simulink model "bataryatermaletkisiz"  (R2020a)
settings: Solver=VariableStepAuto  StartTime=0.0  StopTime=10.0  RelTol=1e-3
undefined symbols (not defined in the file): Ion, Lithium
libraries: electricdrivelib x34, powerlib x5
settings Model: Creator=ASUS  LastModifiedBy=ASUS

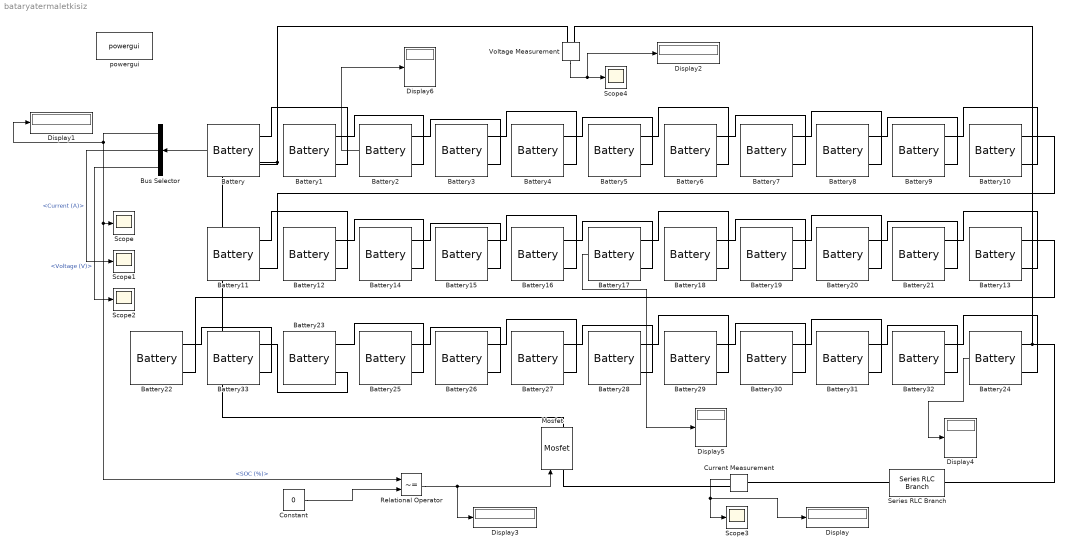
== system bataryatermaletkisiz ==
  Battery{,1..33} (34 alike) : electricdrivelib/Extra Sources/Battery  BatType=Lithium-Ion  ShowTempParam=off  ThermalPreset=no  ShowAgeParam=off  NomV=3.6  NomQ=40.2  SOC=90  Batt_Tr=30  PresetModel=on  MaxQ=40.2  MinV=2.7  FullV=4.1904  Dis_rate=17.4783  R=0.00089552  Normal_OP=36.3548  expZone="[3.8894       1.975]"  current=[6.5 13 32.5]  Units=Time  Tci=20  NomT=20  T2=-30  MaxQ2=4.8  FullV2=7.1  Normal_OP2=5.655  expZone2="[6.58           1]"  Rca=0.6  ti=2000  Dp=0  Neq0=0  Tsim=1e6  Ta1=25  Qeol=5.4*0.9  Reol=0.013333*1.2  Char_age=[2.3478, 3]  Dis_age=[2.3478, 10]  N1=1500  N2=10500  N3=1000  N4=1400  Ta2=45  N5=950
  Bus Selector : BusSelector  OutputSignals=SOC (%),Current (A),Voltage (V)
  Constant : Constant  Value=0
  Current Measurement : powerlib/Measurements/Current Measurement  PhasorSimulation=off  OutputType=Complex  PSBequivalent=0
  Display{,1..6} (7 alike) : Display
  Mosfet : powerlib/Power Electronics/Mosfet  Ron=0.1  Lon=0  Rd=0.01  Vfd=0  IC=0  Rs=1e5  Cs=inf  Measurements=on
  Relational Operator : RelationalOperator  Operator=~=  OutDataTypeStr=boolean  RndMeth=Simplest
  Scope{,1..4} (5 alike) : Scope
  Series RLC Branch : powerlib/Elements/Series RLC Branch  LConnTagsString=__new0  RConnTagsString=__new0  BranchType=R  Resistance=48.4  Inductance=1e-3  SetiL0=off  InitialCurrent=0  Capacitance=1e-6  Setx0=off  InitialVoltage=0  Measurements=None
  Voltage Measurement : powerlib/Measurements/Voltage Measurement  PhasorSimulation=off  OutputType=Complex  PSBequivalent=0
  powergui : powerlib/powergui  Priority=1  SimulationMode=Continuous  SampleTime=50e-6  frequency=60  Iterations=50  frequencyindice=0  Pbase=100e6  ErrMax=1e-4  UnitsV=kV  UnitsW=MW  buscounter=0  FunctionMessages=off  echomessages=off  EnableUseOfTLC=off  CurrentSourceSwitches=off  DisableSnubberDevices=off  DisableRonSwitches=off  DisableVfSwitches=off  DisplayEquations=off  AutomaticDiscreteSolvers=off  SolverType=Tustin/Backward Euler (TBE)  Interpol=off  ExternalGateDelay=off  methode=off  Ts=100  x0status=blocks  SPID=on  SwTol=0  HookPort=off  NonlinearTolerance=1e-4  nMaxIteration=100  ContinueOnMaxIteration=off  RestoreLinks=warning  ResistiveCurrentMeasurement=off  Frange=[0:2:500]  Ylog=off  Xlog=on  ShowGrid=off  save=off  variable=ZData  structure=0  ZoomFFT=off  StartTime=0.0  cycles=1  DisplayStyle=1  fundamental=60  FreqAxis=off  MaxFrequency=1000  frequencyindicesteady=1  RmsSteady=1  display=off
  wires:
  Relational Operator/1 -> Display3/1, Mosfet/1
  Constant/1 -> Relational Operator/2
  Battery/1 -> Bus Selector/1
  Bus Selector/1 -> Display1/1, Relational Operator/1, Scope/1  "<SOC (%)>"
  Bus Selector/2 -> Scope1/1  "<Current (A)>"
  Bus Selector/3 -> Scope2/1  "<Voltage (V)>"
  Current Measurement/1 -> Scope3/1, Display/1
  Voltage Measurement/1 -> Display2/1, Scope4/1
  Battery24/1 -> Display4/1
  Battery17/1 -> Display5/1
  Battery2/1 -> Display6/1
  connections:
  Battery/LConn1 -- Battery1/LConn2
  Battery1/LConn1 -- Battery2/LConn2
  Battery2/LConn1 -- Battery3/LConn2
  Battery3/LConn1 -- Battery4/LConn2
  Battery4/LConn1 -- Battery5/LConn2
  Battery5/LConn1 -- Battery6/LConn2
  Battery6/LConn1 -- Battery7/LConn2
  Battery7/LConn1 -- Battery8/LConn2
  Battery8/LConn1 -- Battery9/LConn2
  Battery9/LConn1 -- Battery10/LConn2
  Battery21/LConn1 -- Battery13/LConn2
  Battery20/LConn1 -- Battery21/LConn2
  Battery16/LConn1 -- Battery17/LConn2
  Battery18/LConn1 -- Battery19/LConn2
  Battery12/LConn1 -- Battery14/LConn2
  Battery14/LConn1 -- Battery15/LConn2
  Battery19/LConn1 -- Battery20/LConn2
  Battery15/LConn1 -- Battery16/LConn2
  Battery17/LConn1 -- Battery18/LConn2
  Battery11/LConn1 -- Battery12/LConn2
  Battery32/LConn1 -- Battery24/LConn2
  Battery31/LConn1 -- Battery32/LConn2
  Battery27/LConn1 -- Battery28/LConn2
  Battery29/LConn1 -- Battery30/LConn2
  Battery23/LConn1 -- Battery25/LConn2
  Battery25/LConn1 -- Battery26/LConn2
  Battery30/LConn1 -- Battery31/LConn2
  Battery26/LConn1 -- Battery27/LConn2
  Battery28/LConn1 -- Battery29/LConn2
  Battery10/LConn1 -- Battery11/LConn2
  Battery13/LConn1 -- Battery22/LConn2
  Current Measurement/LConn1 -- Series RLC Branch/LConn1
  Current Measurement/RConn1 -- Mosfet/LConn1
  Series RLC Branch/RConn1 -- Voltage Measurement/LConn1 -- Battery24/LConn1
  Voltage Measurement/LConn2 -- Mosfet/RConn1 -- Battery/LConn2
  Battery22/LConn1 -- Battery33/LConn2
  Battery33/LConn1 -- Battery23/LConn2
